simulink model "ATOM_simple_planning_simulator"  (R2026a)
settings: Solver=ode4  StopTime=50  FixedStep=0.01
StopFcn:
  | if exist('costmap_active','var') && ...
  |    exist('vehicle','var') && ...
  |    exist('parking_path','var') && ...
  |    ~isempty(parking_path)
  | 
  |     plotPlan(costmap_active, vehicle, parking_path);
  | else
  |     warning('No valid parking path is available for plotting.');
  | end
model workspace (MAT data in the model file):
  vehicle : object (value not decoded)
symbols that are objects in the model workspace (value not decoded): vehicle
undefined symbols (not defined in the file or in its folder): delta_f_LUT, gain4WS_LUT, k_ref_LUT, kappa_gain_BP, Ki, Kp, lateral, longitudinal, planning_validator, rr_gain_BP, rr_LUT, stanley, velocity_smoother
libraries: slpidlib x1, simulink x1
(part 3 of 7)

== matlab function ATOM_simple_planning_simulator/velocity_smoother_node/ApplySteeringRateLimit - velocity_smoother_node/ComputeSteerRateVelocityRatioLimits ==
  data: velocity_thresholds input; steer_rate_velocity_ratio_limits output; steering_angle_rate_limits input
function steer_rate_velocity_ratio_limits = ...
    ComputeSteerRateVelocityRatioLimits( ...
    velocity_thresholds, ...
    steering_angle_rate_limits)

% ComputeSteerRateVelocityRatioLimits
%
% MATLAB equivalent of:
%
%   SmootherBase::computeSteerRateVelocityRatioLimits()
%
% in Autoware.
%
% It computes the steering-rate / velocity ratio limits used later by
% ComputeVelocityLimitFromSteerRate().
%
%
% Equivalent C++:
%
% return computeRatioLimits<double>(
%     velocity_thresholds,
%     steering_angle_rate_limits,
%     compute_steer_rate_ratio);
%
%
% Inputs
% -------
%
% velocity_thresholds
%       Velocity breakpoints [m/s]
%
% steering_angle_rate_limits
%       Maximum steering rate [deg/s]
%
%
% Output
% ------
%
% steer_rate_velocity_ratio_limits
%
% Nx2 matrix equivalent to:
%
% std::vector<std::pair<double,double>>
%
% Each row contains:
%
%   [ratio_lower , ratio_upper]
%
% corresponding to one velocity interval.


epsilon = 1e-5;

N = length(velocity_thresholds);

steer_rate_velocity_ratio_limits = zeros(N+1,2);


%% Compute ratio limits

for i = 1:N

    rate_deg = steering_angle_rate_limits(i);

    vi = velocity_thresholds(i);

    if i == 1
        vi_prev = 0.0;
    else
        vi_prev = velocity_thresholds(i-1);
    end

    steer_rate_velocity_ratio_limits(i,1) = ...
        deg2rad(rate_deg)/(vi_prev + epsilon);

    steer_rate_velocity_ratio_limits(i,2) = ...
        deg2rad(rate_deg)/(vi + epsilon);

end


%% Last interval

v_max = velocity_thresholds(end);

steer_rate_velocity_ratio_limits(end,1) = ...
    deg2rad(steering_angle_rate_limits(end)) / ...
    (v_max + epsilon);

steer_rate_velocity_ratio_limits(end,2) = 0.0;

end

== matlab function ATOM_simple_planning_simulator/velocity_smoother_node/MATLAB Function ==
  data: trajectory_input input; trajectory_output input; curvature input
function PlotSteeringRateVelocityLimit( ...
    trajectory_input, ...
    trajectory_output, ...
    curvature)

% PlotSteeringRateVelocityLimit
%
% Visualizes the velocity modification produced by the steering-rate
% velocity constraint.
%
% Equivalent to inspecting the difference between:
%
%   input.longitudinal_velocity_mps
%
% and:
%
%   output.longitudinal_velocity_mps
%
% after:
%
%   SmootherBase::applySteeringRateLimit()
%
% in Autoware.
%
%
% The steering-rate filter does not modify the trajectory geometry.
% It only reduces longitudinal velocity where the steering rate
% constraint is violated.
%
%
% Inputs
% -------
%
% trajectory_input:
%       Trajectory before ApplySteeringRateVelocityLimit()
%
%       Required fields:
%           trajectory.longitudinal_velocity_mps
%
%
% trajectory_output:
%       Trajectory after ApplySteeringRateVelocityLimit()
%
%       Required fields:
%           trajectory.longitudinal_velocity_mps
%
%
% curvature:
%       trajectory curvature [1/m]
%
%       Used only for visualization of curved regions.
%
%
% Output
% -------
%
% None
%
% Generates diagnostic plots:
%
%   - velocity before/after steering-rate constraint
%   - velocity reduction
%   - curvature profile


%% Extract velocities

vel_in = trajectory_input.longitudinal_velocity_mps;
vel_out = trajectory_output.longitudinal_velocity_mps;


N = length(vel_in);


if length(vel_out) ~= N
    error("Input and output trajectories have different lengths.");
end


%% Velocity variation

velocity_delta = vel_out - vel_in;


%% Plot velocity profile

persistent hVelIn hVelOut hCurvature hVelDelta1 hVelDelta2


if isempty(hVelIn)

    figure(5)
    hold on
    grid on

    hVelIn = plot( ...
        vel_in,...
        'LineWidth',1.5,...
        'DisplayName',"Input velocity");
    
    hVelOut = plot( ...
        vel_out,...
        '--',...
        'LineWidth',1.5,...
        'DisplayName',"After steering-rate limit");


    xlabel("Trajectory point index");
    ylabel("Longitudinal velocity [m/s]");
    
    title("Steering-rate velocity limitation");
    
    legend("Location","best");

else
    
    set(hVelIn, ...
        'YData', vel_in);
    
    set(hVelOut, ...
        'YData', vel_out);
end

%% Plot velocity reduction


if isempty(hVelDelta1)

    figure(6)
    hold on
    grid on

    hVelDelta1 = plot( ...
        velocity_delta,...
        'LineWidth',1.5);
    
    
    yline(0);
    
    
    xlabel("Trajectory point index");
    ylabel("\Delta velocity [m/s]");
    
    
    title("Velocity modification due to steering-rate constraint");

else

    set(hVelDelta1, ...
        'YData', velocity_delta);


end

drawnow limitrate

end

== matlab function ATOM_simple_planning_simulator/Lane Follower Scenario/Demanded trajectory generation: Sinusoid 50m wavelength/Trajectory Generator: sinusoid ==
  data: x output; y output; z output; qx output; qy output; qz output; qw output; longitudinal_velocity_mps output; lateral_velocity_mps output; acceleration_mps2 output; heading_rate_rps output; front_wheel_angle_rad output; rear_wheel_angle_rad output
function [x,y,z,qx,qy,qz,qw,...
    longitudinal_velocity_mps,...
    lateral_velocity_mps,...
    acceleration_mps2,...
    heading_rate_rps,...
    front_wheel_angle_rad,...
    rear_wheel_angle_rad] = trajectoryGenerator

N = 100;

L = 100;                % trajectory length [m]
A = 5;                  % sinusoid amplitude [m]

x = linspace(0,L,N)';
y = A*sin(2*pi*x/50);      % wavelength = 50 m

z = zeros(N,1);

qx = zeros(N,1);
qy = zeros(N,1);
qz = zeros(N,1);
qw = zeros(N,1);

longitudinal_velocity_mps = (8/3.6)*ones(N,1);

lateral_velocity_mps = zeros(N,1);
acceleration_mps2    = zeros(N,1);
heading_rate_rps     = zeros(N,1);

front_wheel_angle_rad = zeros(N,1);
rear_wheel_angle_rad  = zeros(N,1);

%% Orientation

dy = gradient(y,x);

yaw = atan(dy);

qz = sin(yaw/2);
qw = cos(yaw/2);

end

== matlab function ATOM_simple_planning_simulator/Lane Follower Scenario/Demanded trajectory generation: 90° left turn/Trajectory Generator: 90° left turn ==
  data: x output; y output; z output; qx output; qy output; qz output; qw output; longitudinal_velocity_mps output; lateral_velocity_mps output; acceleration_mps2 output; heading_rate_rps output; front_wheel_angle_rad output; rear_wheel_angle_rad output
function [x,y,z,qx,qy,qz,qw,...
          longitudinal_velocity_mps,...
          lateral_velocity_mps,...
          acceleration_mps2,...
          heading_rate_rps,...
          front_wheel_angle_rad,...
          rear_wheel_angle_rad] = trajectoryGenerator

N = 100;

%% Geometry

R = 10;              % curve radius [m]

N1 = 30;            % first straight
N2 = 40;            % circular arc
N3 = 30;            % second straight


%% Allocate outputs

x = zeros(N,1);
y = zeros(N,1);
z = zeros(N,1);

qx = zeros(N,1);
qy = zeros(N,1);
qz = zeros(N,1);
qw = zeros(N,1);

longitudinal_velocity_mps = (15/3.6)*ones(N,1);

lateral_velocity_mps = zeros(N,1);
acceleration_mps2 = zeros(N,1);
heading_rate_rps = zeros(N,1);

front_wheel_angle_rad = zeros(N,1);
rear_wheel_angle_rad = zeros(N,1);


%% ------------------------------------------------------------------------
%% First straight
%% ------------------------------------------------------------------------

L1 = 15;

for i = 1:N1

    t = (i-1)/(N1-1);

    x(i) = t*L1;
    y(i) = 0;

    yaw = 0;

    qz(i) = sin(yaw/2);
    qw(i) = cos(yaw/2);

end


%% ------------------------------------------------------------------------
%% Circular arc (90 deg)
%% ------------------------------------------------------------------------

center_x = L1;
center_y = R;

theta = linspace(-pi/2,0,N2);

for k = 1:N2

    i = N1+k;

    x(i) = center_x + R*cos(theta(k));
    y(i) = center_y + R*sin(theta(k));

    yaw = theta(k)+pi/2;

    qz(i) = sin(yaw/2);
    qw(i) = cos(yaw/2);

end


%% ------------------------------------------------------------------------
%% Second straight
%% ------------------------------------------------------------------------

L2 = 15;

x0 = x(N1+N2);
y0 = y(N1+N2);

for k = 1:N3

    i = N1+N2+k;

    t = k/(N3);

    x(i) = x0;
    y(i) = y0 + t*L2;

    yaw = pi/2;

    qz(i) = sin(yaw/2);
    qw(i) = cos(yaw/2);

end

end

== matlab function ATOM_simple_planning_simulator/trajectory_checker plugin - planning_validator_node/check_valid_steering/calcMaxSteeringAngles/calcSteeringAngles/calcCurvature ==
  data: trajectory input Bus: TrajectoryDataBus; curvature_vector output
function curvature_vector = ComputeTrajectoryCurvaturePlanningValidator(trajectory)

% ComputeTrajectoryCurvaturePlanningValidator
%
% Computes the trajectory curvature exactly as performed by the
% Autoware Planning Validator.
%
% Unlike VelocitySmoother, this implementation does NOT use idx_dist.
%
% Instead, for each trajectory point it searches the first previous and
% next trajectory points located at least:
%
%       curvature_distance = 1.0 [m]
%
% away along the trajectory arc length.
%
% The three selected points are then used by calcCurvature().
%
% This implementation reproduces:
%
% trajectory_checker_utils::calcCurvature()
%
% used inside:
%
% planning_validator
%
%
% Inputs
% -------
%
% trajectory
%
% MATLAB representation of Trajectory.
%
%
% Output
% -------
%
% curvature
%
% Nx1 curvature vector [1/m].

num_points = length(trajectory.pose.position.x);

curvature = zeros(num_points,1);

%% Need at least three points

if num_points < 3
    return
end

%% Arc-length computation

arc_length = zeros(num_points,1);

for i = 2:num_points

    dx = trajectory.pose.position.x(i) - ...
         trajectory.pose.position.x(i-1);

    dy = trajectory.pose.position.y(i) - ...
         trajectory.pose.position.y(i-1);

    ds = hypot(dx,dy);

    arc_length(i) = arc_length(i-1) + ds;

end

%% Curvature computation

curvature_distance = 1.0;      % [m]

first_distant_index = 0;
last_distant_index  = num_points;

for i = 2:num_points-1

    %% Search previous point

    idx_prev = 1;

    for j = i-1:-1:2

        if (arc_length(i)-arc_length(j)) > curvature_distance

            if first_distant_index == 0
                first_distant_index = i;
            end

            idx_prev = j;
            break

        end

    end

    %% Search next point

    idx_next = num_points;

    for j = i+1:num_points-1

        if (arc_length(j)-arc_length(i)) > curvature_distance

            last_distant_index = i;

            idx_next = j;
            break

        end

    end

    %% Extract points

    p1 = [
        trajectory.pose.position.x(idx_prev), ...
        trajectory.pose.position.y(idx_prev), ...
        trajectory.pose.position.z(idx_prev)
        ];

    p2 = [
        trajectory.pose.position.x(i), ...
        trajectory.pose.position.y(i), ...
        trajectory.pose.position.z(i)
        ];

    p3 = [
        trajectory.pose.position.x(idx_next), ...
        trajectory.pose.position.y(idx_next), ...
        trajectory.pose.position.z(idx_next)
        ];

    % In Autoware this call is wrapped inside a try/catch.
    % Since MATLAB code generation does not support exceptions,
    % calcCurvature() is assumed to always return a valid value.
    curvature(i) = calc_curvature(p1,p2,p3);

end

%% Replicate boundary values

% Equivalent to:
%
% for (size_t i = first_distant_index; i > 0; --i)
%   curvature(i-1)=curvature(i);

if first_distant_index > 0

    for i = first_distant_index:-1:2
        curvature(i-1) = curvature(i);
    end

end

% Equivalent to:
%
% for (size_t i = last_distant_index;
%      i < curvature.size()-1;
%      ++i)
%   curvature(i+1)=curvature(i);

if last_distant_index < num_points

    for i = last_distant_index:num_points-1
        curvature(i+1) = curvature(i);
    end

end

curvature_vector = curvature;

end

== matlab function ATOM_simple_planning_simulator/trajectory_checker plugin - planning_validator_node/check_valid_steering/calcMaxSteeringAngles/calcSteeringAngles/steering_vector calculation ==
  data: curvature input; front_steering_vector output; rear_steering_vector output; veh input
function [front_steering_vector, rear_steering_vector] = calcSteeringVector(curvature, veh)

wheel_base = veh(3);
rear_steering_ratio = veh(29);

N = length(curvature);

front_steering_vector = zeros(N,1);
rear_steering_vector  = zeros(N,1);

for i = 1:N

    front_steering_vector(i) = ...
        CalculateFrontSteeringAngle4WS( ...
        curvature(i),...
        wheel_base,...
        rear_steering_ratio);

    rear_steering_vector(i) = rear_steering_ratio*front_steering_vector(i);
    
end
    
end

== matlab function ATOM_simple_planning_simulator/trajectory_checker plugin - planning_validator_node/check_valid_steering/calcMaxSteeringAngles/GetAbsMaxValAndIdx front ==
  data: values input; max_value output; max_index output
function [max_value, max_index] = GetAbsMaxValAndIdx(values)

% GetAbsMaxValAndIdx
%
% Returns the maximum absolute value contained in the input vector and
% its corresponding index.
%
% Equivalent to:
%
% trajectory_checker_utils::getAbsMaxValAndIdx()
%
% in Autoware.
%
% C++ implementation:
%
% std::pair<double, size_t> getAbsMaxValAndIdx(...)
%
% which internally uses:
%
%   std::max_element(...)
%
% with the comparison:
%
%   abs(a) < abs(b)
%
%
% Inputs
% -------
%
% values
%     Nx1 vector.
%
%
% Outputs
% --------
%
% max_value
%     Maximum absolute value contained in the vector.
%
% max_index
%     Index of the element whose absolute value is maximum.
%
% Note
% ----
%
% MATLAB indices are 1-based, whereas the equivalent C++ implementation
% returns a 0-based index.

[max_value, max_index] = max(abs(values));

end

== matlab function ATOM_simple_planning_simulator/trajectory_checker plugin - planning_validator_node/check_valid_steering/calcMaxSteeringAngles/GetAbsMaxValAndIdx rear ==
  data: values input; max_value output; max_index output
function [max_value, max_index] = GetAbsMaxValAndIdx(values)

% GetAbsMaxValAndIdx
%
% Returns the maximum absolute value contained in the input vector and
% its corresponding index.
%
% Equivalent to:
%
% trajectory_checker_utils::getAbsMaxValAndIdx()
%
% in Autoware.
%
% C++ implementation:
%
% std::pair<double, size_t> getAbsMaxValAndIdx(...)
%
% which internally uses:
%
%   std::max_element(...)
%
% with the comparison:
%
%   abs(a) < abs(b)
%
%
% Inputs
% -------
%
% values
%     Nx1 vector.
%
%
% Outputs
% --------
%
% max_value
%     Maximum absolute value contained in the vector.
%
% max_index
%     Index of the element whose absolute value is maximum.
%
% Note
% ----
%
% MATLAB indices are 1-based, whereas the equivalent C++ implementation
% returns a 0-based index.

[max_value, max_index] = max(abs(values));

end

== matlab function ATOM_simple_planning_simulator/trajectory_checker plugin - planning_validator_node/check_valid_steering/calcMaxSteeringAngles/DecideValIdx ==
  data: max_steering output; max_index output; max_front input; idx_front input; max_rear input; idx_rear input
function [max_steering, max_index] = DecideValIdx(max_front, idx_front, ...
                                                  max_rear, idx_rear) 


if max_front >= max_rear

    max_steering = max_front;
    max_index    = idx_front;

else

    max_steering = max_rear;
    max_index    = idx_rear;

end

end

== matlab function ATOM_simple_planning_simulator/trajectory_checker plugin - planning_validator_node/check_valid_steering/CheckValidSteering ==
  data: max_steering input; is_valid_steering output; steering_threshold input
function is_valid_steering  = ...
    CheckValidSteering4WS( ...
    max_steering, steering_threshold)


% CheckValidSteering4WS
%
% Equivalent to:
%
% TrajectoryChecker::check_valid_steering()
%
% Autoware planning_validator
%
%
% The steering angle is NOT taken from:
%
%   trajectory.front_wheel_angle_rad
%   trajectory.rear_wheel_angle_rad
%
% Instead, Autoware recomputes it from trajectory geometry:
%
%   trajectory
%        |
%        v
%   curvature_vector
%        |
%        v
%   steering angle
%
%
% Adapted for 4WS:
%
% curvature =
%
%       (tan(delta_f)-tan(delta_r))/L
%
%
% where:
%
%       delta_r = rear_steering_ratio * delta_f
%
%
% Inputs
% -------
%
% trajectory:
%
%   trajectory.pose.position.x
%   trajectory.pose.position.y
%
%
% wheel_base:
%
%   vehicle wheelbase [m]
%
%
% rear_steering_ratio:
%
%   rear/front steering ratio
%
%
% steering_threshold:
%
%   maximum allowed steering angle [rad]
%
%
%
% Outputs
% --------
%
% is_valid_steering:
%
%   true  -> steering OK
%   false -> steering violation
%
%
% max_steering:
%
%   maximum absolute steering angle [rad]
%
%
% max_index:
%
%   trajectory point where maximum steering occurs
%
%
%

%% ============================================================
% Equivalent to:
%
% if (max_steering > params_.steering.threshold)
%
% =============================================================


if max_steering > steering_threshold

    is_valid_steering = false;

else

    is_valid_steering = true;

end


end

== matlab function ATOM_simple_planning_simulator/trajectory_checker plugin - planning_validator_node/check_valid_steering_rate/CheckValidSteeringRate ==
  data: max_steering_rate input; is_valid_steering_rate output; steering_rate_threshold input
function is_valid_steering_rate  = ...
    CheckValidSteering4WS( ...
    max_steering_rate, steering_rate_threshold)


% CheckValidSteering4WS
%
% Equivalent to:
%
% TrajectoryChecker::check_valid_steering()
%
% Autoware planning_validator
%
%
% The steering angle is NOT taken from:
%
%   trajectory.front_wheel_angle_rad
%   trajectory.rear_wheel_angle_rad
%
% Instead, Autoware recomputes it from trajectory geometry:
%
%   trajectory
%        |
%        v
%   curvature_vector
%        |
%        v
%   steering angle
%
%
% Adapted for 4WS:
%
% curvature =
%
%       (tan(delta_f)-tan(delta_r))/L
%
%
% where:
%
%       delta_r = rear_steering_ratio * delta_f
%
%
% Inputs
% -------
%
% trajectory:
%
%   trajectory.pose.position.x
%   trajectory.pose.position.y
%
%
% wheel_base:
%
%   vehicle wheelbase [m]
%
%
% rear_steering_ratio:
%
%   rear/front steering ratio
%
%
% steering_threshold:
%
%   maximum allowed steering angle [rad]
%
%
%
% Outputs
% --------
%
% is_valid_steering:
%
%   true  -> steering OK
%   false -> steering violation
%
%
% max_steering:
%
%   maximum absolute steering angle [rad]
%
%
% max_index:
%
%   trajectory point where maximum steering occurs
%
%
%

%% ============================================================
% Equivalent to:
%
% if (max_steering > params_.steering.threshold)
%
% =============================================================


if max_steering_rate > steering_rate_threshold

    is_valid_steering_rate = false;

else

    is_valid_steering_rate = true;

end


end

== matlab function ATOM_simple_planning_simulator/trajectory_checker plugin - planning_validator_node/check_valid_steering_rate/calcMaxSteeringRates/DecideValIdx ==
  data: max_steering_rate output; max_index output; max_front input; idx_front input; max_rear input; idx_rear input
function [max_steering_rate, max_index] = DecideValIdx(max_front, idx_front, ...
                                                  max_rear, idx_rear) 


if max_front >= max_rear

    max_steering_rate = max_front;
    max_index    = idx_front;

else

    max_steering_rate = max_rear;
    max_index    = idx_rear;

end

end

== matlab function ATOM_simple_planning_simulator/trajectory_checker plugin - planning_validator_node/check_valid_steering_rate/calcMaxSteeringRates/MATLAB Function ==
  data: trajectory input; max_steering_rate output; steering_vector input; max_index output
function [max_steering_rate, max_index] = ...
    CalcMaxSteeringRate(trajectory, steering_vector)


% CalcMaxSteeringRate
%
% Equivalent to:
%
% trajectory_checker_utils::calcMaxSteeringRates()
%
% in Autoware planning_validator.
%
%
% For 2WS:
%   steering_vector = front steering angle
%
% For 4WS:
%   call this function twice:
%
%   front_rate = CalcMaxSteeringRate(trajectory, front_vector)
%   rear_rate  = CalcMaxSteeringRate(trajectory, rear_vector)
%
% and take:
%
%   max(front_rate,rear_rate)
%
%
% Steering rate:
%
%       d(delta)/dt
%
% where:
%
%       dt = delta_s / velocity
%
%
% Units:
%
% steering_vector : [rad]
% trajectory velocity : [m/s]
% output : [rad/s]


N = length(steering_vector);


if N < 2

    max_steering_rate = 0;
    max_index = 1;

    return

end


max_steering_rate = 0;
max_index = 1;



for i = 1:N-1


    %% Distance between trajectory points

    dx = trajectory.pose.position.x(i+1) - ...
         trajectory.pose.position.x(i);

    dy = trajectory.pose.position.y(i+1) - ...
         trajectory.pose.position.y(i);


    delta_s = sqrt(dx^2 + dy^2);



    %% Mean velocity

    v = 0.5 * ( ...
        trajectory.longitudinal_velocity_mps(i+1) + ...
        trajectory.longitudinal_velocity_mps(i));



    %% Equivalent of:
    %
    % delta_s / max(v,1e-5)
    %
    % in C++

    dt = delta_s / max(v,1e-5);



    %% Steering rate

    steer_rate = ...
        (steering_vector(i+1)-steering_vector(i)) / dt;



    %% Equivalent of takeBigger()

    if abs(steer_rate) > max_steering_rate

        max_steering_rate = abs(steer_rate);

        max_index = i;

    end

end


end

== matlab function ATOM_simple_planning_simulator/trajectory_checker plugin - planning_validator_node/check_valid_steering_rate/calcMaxSteeringRates/MATLAB Function1 ==
  data: trajectory input; max_steering_rate output; steering_vector input; max_index output
function [max_steering_rate, max_index] = ...
    CalcMaxSteeringRate(trajectory, steering_vector)


% CalcMaxSteeringRate
%
% Equivalent to:
%
% trajectory_checker_utils::calcMaxSteeringRates()
%
% in Autoware planning_validator.
%
%
% For 2WS:
%   steering_vector = front steering angle
%
% For 4WS:
%   call this function twice:
%
%   front_rate = CalcMaxSteeringRate(trajectory, front_vector)
%   rear_rate  = CalcMaxSteeringRate(trajectory, rear_vector)
%
% and take:
%
%   max(front_rate,rear_rate)
%
%
% Steering rate:
%
%       d(delta)/dt
%
% where:
%
%       dt = delta_s / velocity
%
%
% Units:
%
% steering_vector : [rad]
% trajectory velocity : [m/s]
% output : [rad/s]


N = length(steering_vector);


if N < 2

    max_steering_rate = 0;
    max_index = 1;

    return

end


max_steering_rate = 0;
max_index = 1;



for i = 1:N-1


    %% Distance between trajectory points

    dx = trajectory.pose.position.x(i+1) - ...
         trajectory.pose.position.x(i);

    dy = trajectory.pose.position.y(i+1) - ...
         trajectory.pose.position.y(i);


    delta_s = sqrt(dx^2 + dy^2);



    %% Mean velocity

    v = 0.5 * ( ...
        trajectory.longitudinal_velocity_mps(i+1) + ...
        trajectory.longitudinal_velocity_mps(i));



    %% Equivalent of:
    %
    % delta_s / max(v,1e-5)
    %
    % in C++

    dt = delta_s / max(v,1e-5);



    %% Steering rate

    steer_rate = ...
        (steering_vector(i+1)-steering_vector(i)) / dt;



    %% Equivalent of takeBigger()

    if abs(steer_rate) > max_steering_rate

        max_steering_rate = abs(steer_rate);

        max_index = i;

    end

end


end

== matlab function ATOM_simple_planning_simulator/trajectory_checker plugin - planning_validator_node/check_valid_steering_rate/calcMaxSteeringRates/calcSteeringAngles/calcCurvature ==
  data: trajectory input Bus: TrajectoryDataBus; curvature_vector output
function curvature_vector = ComputeTrajectoryCurvaturePlanningValidator(trajectory)

% ComputeTrajectoryCurvaturePlanningValidator
%
% Computes the trajectory curvature exactly as performed by the
% Autoware Planning Validator.
%
% Unlike VelocitySmoother, this implementation does NOT use idx_dist.
%
% Instead, for each trajectory point it searches the first previous and
% next trajectory points located at least:
%
%       curvature_distance = 1.0 [m]
%
% away along the trajectory arc length.
%
% The three selected points are then used by calcCurvature().
%
% This implementation reproduces:
%
% trajectory_checker_utils::calcCurvature()
%
% used inside:
%
% planning_validator
%
%
% Inputs
% -------
%
% trajectory
%
% MATLAB representation of Trajectory.
%
%
% Output
% -------
%
% curvature
%
% Nx1 curvature vector [1/m].

num_points = length(trajectory.pose.position.x);

curvature = zeros(num_points,1);

%% Need at least three points

if num_points < 3
    return
end

%% Arc-length computation

arc_length = zeros(num_points,1);

for i = 2:num_points

    dx = trajectory.pose.position.x(i) - ...
         trajectory.pose.position.x(i-1);

    dy = trajectory.pose.position.y(i) - ...
         trajectory.pose.position.y(i-1);

    ds = hypot(dx,dy);

    arc_length(i) = arc_length(i-1) + ds;

end

%% Curvature computation

curvature_distance = 1.0;      % [m]

first_distant_index = 0;
last_distant_index  = num_points;

for i = 2:num_points-1

    %% Search previous point

    idx_prev = 1;

    for j = i-1:-1:2

        if (arc_length(i)-arc_length(j)) > curvature_distance

            if first_distant_index == 0
                first_distant_index = i;
            end

            idx_prev = j;
            break

        end

    end

    %% Search next point

    idx_next = num_points;

    for j = i+1:num_points-1

        if (arc_length(j)-arc_length(i)) > curvature_distance

            last_distant_index = i;

            idx_next = j;
            break

        end

    end

    %% Extract points

    p1 = [
        trajectory.pose.position.x(idx_prev), ...
        trajectory.pose.position.y(idx_prev), ...
        trajectory.pose.position.z(idx_prev)
        ];

    p2 = [
        trajectory.pose.position.x(i), ...
        trajectory.pose.position.y(i), ...
        trajectory.pose.position.z(i)
        ];

    p3 = [
        trajectory.pose.position.x(idx_next), ...
        trajectory.pose.position.y(idx_next), ...
        trajectory.pose.position.z(idx_next)
        ];

    % In Autoware this call is wrapped inside a try/catch.
    % Since MATLAB code generation does not support exceptions,
    % calcCurvature() is assumed to always return a valid value.
    curvature(i) = calc_curvature(p1,p2,p3);

end

%% Replicate boundary values

% Equivalent to:
%
% for (size_t i = first_distant_index; i > 0; --i)
%   curvature(i-1)=curvature(i);

if first_distant_index > 0

    for i = first_distant_index:-1:2
        curvature(i-1) = curvature(i);
    end

end

% Equivalent to:
%
% for (size_t i = last_distant_index;
%      i < curvature.size()-1;
%      ++i)
%   curvature(i+1)=curvature(i);

if last_distant_index < num_points

    for i = last_distant_index:num_points-1
        curvature(i+1) = curvature(i);
    end

end

curvature_vector = curvature;

end

== matlab function ATOM_simple_planning_simulator/trajectory_checker plugin - planning_validator_node/check_valid_steering_rate/calcMaxSteeringRates/calcSteeringAngles/steering_vector calculation ==
  data: curvature input; front_steering_vector output; rear_steering_vector output; veh input
function [front_steering_vector, rear_steering_vector] = calcSteeringVector(curvature, veh)

wheel_base = veh(3);
rear_steering_ratio = veh(29);

N = length(curvature);

front_steering_vector = zeros(N,1);
rear_steering_vector  = zeros(N,1);

for i = 1:N

    front_steering_vector(i) = ...
        CalculateFrontSteeringAngle4WS( ...
        curvature(i),...
        wheel_base,...
        rear_steering_ratio);

    rear_steering_vector(i) = rear_steering_ratio*front_steering_vector(i);
    
end
    
end

== matlab function ATOM_simple_planning_simulator/trajectory_checker plugin - planning_validator_node/HandleInvalidTrajectory - handling_type == default (case 0) ==
  data: trajectory_in input Bus: TrajectoryDataBus; trajectory_out output Bus: TrajectoryDataBus; is_valid_steering input; is_valid_steering_rate input
function trajectory_out  = ...
    HandleInvalidTrajectory( ...
    trajectory_in, ...
    is_valid_steering, ...
    is_valid_steering_rate)


% HandleInvalidTrajectory
%
% Equivalent to:
%
% PlanningValidatorNode::publishTrajectory()
%
% when:
%
% InvalidTrajectoryHandlingType::PUBLISH_AS_IT_IS
%
%
% If validation fails:
%
%   - trajectory is published unchanged
%   - validation status reports failure
%   - caution message is generated
%
%
% This reproduces Autoware behaviour.


%% ============================================================
% Validation status
% =============================================================

validation_status = ...
    is_valid_steering && is_valid_steering_rate;



%% ============================================================
% Publish trajectory behaviour
% =============================================================

% Default behaviour:
%
% PUBLISH_AS_IT_IS
%
% Therefore:
%
% output trajectory = input trajectory


trajectory_out = trajectory_in;



%% ============================================================
% Warning message
% =============================================================


if validation_status == false

     warning("Caution! Invalid Trajectory published.")

end


end

== matlab function ATOM_simple_planning_simulator/Lane Follower Scenario/Demanded trajectory generation: 90° left turn critical for 2WS --> R = 2.5 m/Trajectory Generator: 90° left turn critical for 2WS ==
  data: x output; y output; z output; qx output; qy output; qz output; qw output; longitudinal_velocity_mps output; lateral_velocity_mps output; acceleration_mps2 output; heading_rate_rps output; front_wheel_angle_rad output; rear_wheel_angle_rad output
function [x,y,z,qx,qy,qz,qw,...
          longitudinal_velocity_mps,...
          lateral_velocity_mps,...
          acceleration_mps2,...
          heading_rate_rps,...
          front_wheel_angle_rad,...
          rear_wheel_angle_rad] = trajectoryGenerator

N = 100;

%% Geometry

R = 1;              % curve radius [m]

N1 = 30;            % first straight
N2 = 40;            % circular arc
N3 = 30;            % second straight


%% Allocate outputs

x = zeros(N,1);
y = zeros(N,1);
z = zeros(N,1);

qx = zeros(N,1);
qy = zeros(N,1);
qz = zeros(N,1);
qw = zeros(N,1);

longitudinal_velocity_mps = (4/3.6)*ones(N,1);

lateral_velocity_mps = zeros(N,1);
acceleration_mps2 = zeros(N,1);
heading_rate_rps = zeros(N,1);

front_wheel_angle_rad = zeros(N,1);
rear_wheel_angle_rad = zeros(N,1);


%% ------------------------------------------------------------------------
%% First straight
%% ------------------------------------------------------------------------

L1 = 2;

for i = 1:N1

    t = (i-1)/(N1-1);

    x(i) = t*L1;
    y(i) = 0;

    yaw = 0;

    qz(i) = sin(yaw/2);
    qw(i) = cos(yaw/2);

end


%% ------------------------------------------------------------------------
%% Circular arc (90 deg)
%% ------------------------------------------------------------------------

center_x = L1;
center_y = R;

theta = linspace(-pi/2,0,N2);

for k = 1:N2

    i = N1+k;

    x(i) = center_x + R*cos(theta(k));
    y(i) = center_y + R*sin(theta(k));

    yaw = theta(k)+pi/2;

    qz(i) = sin(yaw/2);
    qw(i) = cos(yaw/2);

end


%% ------------------------------------------------------------------------
%% Second straight
%% ------------------------------------------------------------------------

L2 = 15;

x0 = x(N1+N2);
y0 = y(N1+N2);

for k = 1:N3

    i = N1+N2+k;

    t = k/(N3);

    x(i) = x0;
    y(i) = y0 + t*L2;

    yaw = pi/2;

    qz(i) = sin(yaw/2);
    qw(i) = cos(yaw/2);

end

end

== matlab function ATOM_simple_planning_simulator/Lateral run()/RearToFrontOdometry ==
  data: rear_pose input Bus: KinematicStateBus; front_pose_pred output Bus: KinematicStateBus; wheel_base input; tau_max input; d0 input; k_preview input
function front_pose_pred = RearToFrontOdometryPredictive( ...
    rear_pose,...
    wheel_base,...
    tau_max,...
    d0, k_preview)

%% ============================================================
% Predictive Rear -> Front transformation
%
% Position preview:
%   compensates steering actuator delay
%
% Orientation preview:
%   reduced anticipation for Stanley heading error
%
%% ============================================================


%% Preview times

vx = max(abs(rear_pose.twist.linear.x),0.1);

tau_pos = min(tau_max,d0/vx);

tau_yaw = k_preview*tau_pos;



%% Current rear axle state

x_r = rear_pose.pose.position.x;
y_r = rear_pose.pose.position.y;

qx = rear_pose.pose.orientation.x;
qy = rear_pose.pose.orientation.y;
qz = rear_pose.pose.orientation.z;
qw = rear_pose.pose.orientation.w;

yaw = QuaternionToYaw(qx,qy,qz,qw);



%% Vehicle velocities (body frame)

vx_body = rear_pose.twist.linear.x;
vy_body = rear_pose.twist.linear.y;

yaw_rate = rear_pose.twist.angular.z;



%% Body -> World

vx_world = ...
    vx_body*cos(yaw) - ...
    vy_body*sin(yaw);

vy_world = ...
    vx_body*sin(yaw) + ...
    vy_body*cos(yaw);



%% ============================================================
% Predict rear axle position
%% ============================================================

x_r_pred = x_r + vx_world*tau_pos;

y_r_pred = y_r + vy_world*tau_pos;



%% Orientation previews

yaw_pos  = yaw + yaw_rate*tau_pos;

yaw_ctrl = yaw + yaw_rate*tau_yaw;



%% ============================================================
% Predicted front axle position
%% ============================================================

x_f_pred = ...
    x_r_pred + wheel_base*cos(yaw_pos);

y_f_pred = ...
    y_r_pred + wheel_base*sin(yaw_pos);



%% Output

front_pose_pred = rear_pose;

front_pose_pred.pose.position.x = x_f_pred;
front_pose_pred.pose.position.y = y_f_pred;
front_pose_pred.pose.position.z = rear_pose.pose.position.z;


[qx,qy,qz,qw] = yawToQuaternion(yaw_ctrl);

front_pose_pred.pose.orientation.x = qx;
front_pose_pred.pose.orientation.y = qy;
front_pose_pred.pose.orientation.z = qz;
front_pose_pred.pose.orientation.w = qw;



%% Predicted front axle velocity (body frame)

front_pose_pred.twist.linear.x = vx_body;

front_pose_pred.twist.linear.y = ...
    vy_body + yaw_rate*wheel_base;

front_pose_pred.twist.linear.z = rear_pose.twist.linear.z;

end

== matlab function ATOM_simple_planning_simulator/Lateral run()/SetStanleyTrajectory/Resample Trajectory ==
  data: trajectory_in input Bus: TrajectoryDataBus; trajectory_out output Bus: TrajectoryDataBus; resample_interval_dist input; nearest_seg_idx input; ego_offset_to_segment input
function trajectory_out = resampleTrajectoryByDistance( ...
    trajectory_in, ...
    resample_interval_dist, ...
    nearest_seg_idx, ...
    ego_offset_to_segment)


%% ============================================================
% RESAMPLE TRAJECTORY BY ARC LENGTH
%
% Equivalent to:
%
% MPCUtils::resampleMPCTrajectoryByDistance()
%
% Adapted for Stanley controller.
%
% Unlike MPC:
% - no MPCTrajectory conversion
% - no curvature resampling
% - no optimization variables
%
% The trajectory is directly interpolated in arc length.
%
% ATTENTION:
% 
% Resampling is not actuated in Simulink since in/out buses present fixed sizes.
% See NOTE at the end of this function.
%
% =============================================================


% N = length(trajectory_in.pose.position.x);
% 
% 
% if N < 2
% 
%     trajectory_out = trajectory_in;
%     return
% 
% end
% 
% 
% 
% %% ============================================================
% % Compute arc length
% % =============================================================
% 
% x = trajectory_in.pose.position.x;
% y = trajectory_in.pose.position.y;
% 
% 
% arc_length = zeros(N,1);
% 
% 
% for i = 2:N
% 
%     dx = x(i)-x(i-1);
%     dy = y(i)-y(i-1);
% 
%     arc_length(i)= ...
%         arc_length(i-1)+sqrt(dx^2+dy^2);
% 
% end
% 
% 
% 
% if isempty(arc_length)
% 
%     trajectory_out = trajectory_in;
%     return
% 
% end
% 
% 
% 
% %% ============================================================
% % Ego position along trajectory
% %
% % Equivalent to:
% %
% % input_arclength(nearest_seg_idx)
% % + ego_offset_to_segment
% %
% % =============================================================
% 
% 
% ego_s = arc_length(nearest_seg_idx) ...
%         + ego_offset_to_segment;
% 
% 
% ego_s = min(max(ego_s,0),arc_length(end));
% 
% 
% 
% %% ============================================================
% % Generate resampling points
% %
% % Same strategy as Autoware:
% % - backward from ego
% % - forward from ego
% %
% % =============================================================
% 
% 
% output_s = [];
% 
% 
% % backward direction
% 
% s = ego_s;
% 
% while s >= 0
% 
%     output_s = [s output_s]; %#ok<AGROW>
% 
%     s = s - resample_interval_dist;
% 
% end
% 
% 
% 
% % forward direction
% 
% s = ego_s + resample_interval_dist;
% 
% 
% while s < arc_length(end)
% 
%     output_s(end+1)=s; % #ok<AGROW>
% 
%     s = s + resample_interval_dist;
% 
% end
% 
% 
% 
% %% ============================================================
% % Interpolation
% % =============================================================
% 
% 
% x_new = interp1( ...
%     arc_length,...
%     x,...
%     output_s,...
%     'linear');
% 
% 
% 
% y_new = interp1( ...
%     arc_length,...
%     y,...
%     output_s,...
%     'linear');
% 
% 
% 
% z = trajectory_in.pose.position.z;
% 
% z_new = interp1( ...
%     arc_length,...
%     z,...
%     output_s,...
%     'linear');
% 
% 
% 
% %% ============================================================
% % Quaternion / yaw interpolation
% %
% % Stanley works with yaw.
% % Therefore interpolate yaw and rebuild quaternion.
% %
% % =============================================================
% 
% 
% yaw = QuaternionToYaw( ...
%     trajectory_in.pose.orientation.qx,...
%     trajectory_in.pose.orientation.qy,...
%     trajectory_in.pose.orientation.qz,...
%     trajectory_in.pose.orientation.qw);
% 
% 
% 
% % avoid discontinuity
% 
% yaw = unwrap(yaw);
% 
% 
% 
% yaw_new = interp1( ...
%     arc_length,...
%     yaw,...
%     output_s,...
%     'linear');
% 
% 
% 
% %% ============================================================
% % Velocity interpolation
% %
% % Autoware uses linear interpolation
% % =============================================================
% 
% 
% vel_new = interp1( ...
%     arc_length,...
%     trajectory_in.longitudinal_velocity_mps,...
%     output_s,...
%     'linear');
% 
% 
% 
% lat_vel_new = interp1( ...
%     arc_length,...
%     trajectory_in.lateral_velocity_mps,...
%     output_s,...
%     'linear');
% 
% 
% 
% acc_new = interp1( ...
%     arc_length,...
%     trajectory_in.acceleration_mps2,...
%     output_s,...
%     'linear');
% 
% 
% 
% %% ============================================================
% % Build output structure
% % =============================================================
% 
% 
% M = length(output_s);
% 
% 
% trajectory_out.pose.position.x = x_new;
% trajectory_out.pose.position.y = y_new;
% trajectory_out.pose.position.z = z_new;
% 
% 
% 
% [qx,qy,qz,qw] = yawToQuaternion(yaw_new);
% 
% 
% 
% trajectory_out.pose.orientation.qx = qx;
% trajectory_out.pose.orientation.qy = qy;
% trajectory_out.pose.orientation.qz = qz;
% trajectory_out.pose.orientation.qw = qw;
% 
% 
% 
% trajectory_out.longitudinal_velocity_mps = vel_new;
% 
% trajectory_out.lateral_velocity_mps = lat_vel_new;
% 
% trajectory_out.acceleration_mps2 = acc_new;
% 
% 
% 
% % steering values are kept
% 
% trajectory_out.front_wheel_angle_rad = ...
%     interp1( ...
%     arc_length,...
%     trajectory_in.front_wheel_angle_rad,...
%     output_s,...
%     'linear');
% 
% 
% trajectory_out.rear_wheel_angle_rad = ...
%     interp1( ...
%     arc_length,...
%     trajectory_in.rear_wheel_angle_rad,...
%     output_s,...
%     'linear');
% 
% 


%% ============================================================
% NOTE (Simulink Implementation)
%
% The trajectory resampling algorithm reported above is equivalent
% to the implementation adopted by Autoware.
%
% However, the main objective of the present work is the development
% and validation of the 4WS Stanley Controller rather than the
% trajectory preprocessing module.
%
% Since Simulink requires fixed-size bus signals, the resampled
% trajectory is not generated in the simulation model.
%
% The original input trajectory is therefore directly propagated to
% the controller, preserving its fixed dimension and avoiding the
% introduction of variable-length signals.
%
% Consequently, the following assignment overwrites the resampled
% trajectory computed above.
%
% ============================================================

trajectory_out = trajectory_in;

end

== matlab function ATOM_simple_planning_simulator/LongitudinalRun()/RearToFrontOdometry ==
  data: rear_pose input Bus: KinematicStateBus; front_pose_pred output Bus: KinematicStateBus; wheel_base input
function front_pose_pred = RearToFrontOdometryCurrent( ...
    rear_pose, ...
    wheel_base)

front_pose_pred = rear_pose;

% 1. Estrazione dello Yaw dall'orientamento (Quaternion -> Yaw)
qx = rear_pose.pose.orientation.x;
qy = rear_pose.pose.orientation.y;
qz = rear_pose.pose.orientation.z;
qw = rear_pose.pose.orientation.w;
yaw = QuaternionToYaw(qx, qy, qz, qw);

% 2. Calcolo della Posizione Attuale dell'Asse Anteriore (Mappa/World Frame)
x_front_now = rear_pose.pose.position.x + wheel_base * cos(yaw);
y_front_now = rear_pose.pose.position.y + wheel_base * sin(yaw);

% 3. Velocità dell'Asse Anteriore espresso nel Frame Veicolo (Body Frame)
v_x_body = rear_pose.twist.linear.x;
v_y_body = rear_pose.twist.linear.y + rear_pose.twist.angular.z * wheel_base;

% 4. Conversione delle Velocità dal Frame Veicolo (Body) al Frame Mappa (World)
% Ruotiamo il vettore velocità [v_x_body, v_y_body] dell'angolo yaw attuale:
v_x_world = v_x_body * cos(yaw) - v_y_body * sin(yaw);
v_y_world = v_x_body * sin(yaw) + v_y_body * cos(yaw);

% 5. PREDIZIONE TEMPORALE (Coordinate t + tau nel Frame Mappa)
front_pose_pred.pose.position.x = x_front_now;
front_pose_pred.pose.position.y = y_front_now;
front_pose_pred.pose.position.z = rear_pose.pose.position.z;

% 6. Aggiornamento delle velocità nel messaggio di output (Frame Veicolo)
front_pose_pred.twist.linear.x = v_x_body;
front_pose_pred.twist.linear.y = v_y_body;
front_pose_pred.twist.linear.z = rear_pose.twist.linear.z;

% 7. L'orientamento rimane lo stesso (o aggiornato con il pitch/roll se presente)
front_pose_pred.pose.orientation = rear_pose.pose.orientation;

end

== matlab function ATOM_simple_planning_simulator/Lateral run()/SetStanleyTrajectory/calcLongOffsetToSegment ==
  data: seg_idx input; ego_pose input; trajectory input Bus: TrajectoryDataBus; ego_offset_to_segment output
function ego_offset_to_segment = calcLongOffsetToSegment(seg_idx, ego_pose, trajectory)

ego_offset_to_segment = calcLongitudinalOffsetToSegment(trajectory, seg_idx, ego_pose);

end

== matlab function ATOM_simple_planning_simulator/Lateral run()/SetStanleyTrajectory/findFirstNearestSegmentIndexWithSoftConstraints ==
  data: trajectory input; dist_threshold input; yaw_threshold input; nearest_seg_idx output; pose input
function nearest_seg_idx = findNearestSegmentIndexWithSoftConstraints( ...
    trajectory, dist_threshold, yaw_threshold, pose)


%% Step 1:
% Find nearest point index

nearest_idx = findFirstNearestIndexWithSoftConstraints( ...
    trajectory, ...
    pose, ...
    dist_threshold, ...
    yaw_threshold);


N = length(trajectory.pose.position.x);


%% Step 2:
% Convert point index into segment index

% First point
if nearest_idx == 1

    nearest_seg_idx = 1;
    return

end


% Last point
if nearest_idx == N

    nearest_seg_idx = N-1;
    return

end



%% Step 3:
% Determine whether ego lies before or after nearest point
%
% Equivalent to Autoware:
%
% signed_length =
% calcLongitudinalOffsetToSegment(points,
%                                 nearest_idx,
%                                 pose.position)


signed_length = calcLongitudinalOffsetToSegment( ...
    trajectory,...
    nearest_idx,...
    pose);



%% Step 4:
% Choose segment

if signed_length <= 0

    % ego is before nearest point
    %
    % Autoware:
    % return nearest_idx - 1;

    nearest_seg_idx = nearest_idx - 1;


else

    % ego is after nearest point
    %
    % Autoware:
    % return nearest_idx;

    nearest_seg_idx = nearest_idx;

end


end

== matlab function ATOM_simple_planning_simulator/Lateral run()/MATLAB Function ==
  data: offset_limit input; enable_offset_removal input; steering_offset input; offset output
function offset = getSteeringOffset(offset_limit, enable_offset_removal, steering_offset)

persistent current_offset
if isempty(current_offset)
    current_offset = 0;
end

if enable_offset_removal
    current_offset = steering_offset;
end

offset = min(max(current_offset, -offset_limit), offset_limit);
